simulink model "Problem8"  (R2020b)
settings: Solver=VariableStepAuto  StartTime=0.0  StopTime=inf  RelTol=1e-3
settings Model: Creator=Dell  LastModifiedBy=Dell

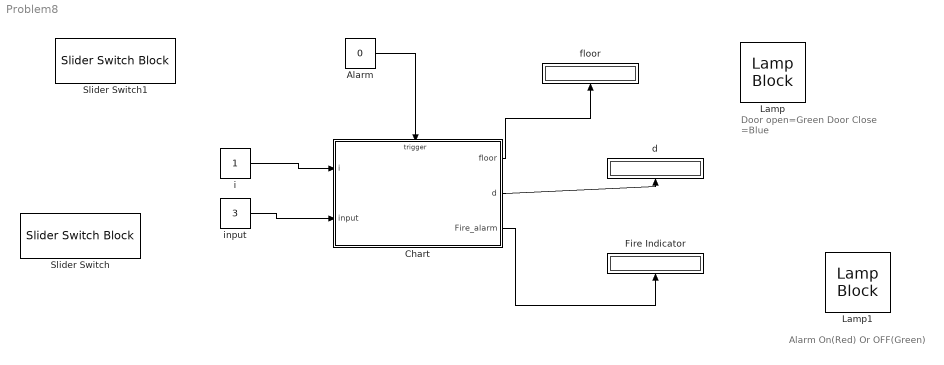
== system Problem8 ==
  note: Alarm On(Red) Or OFF(Green)
  note: Door open=Green
      | Door Close =Blue
  Alarm : Constant  Value=0
  Chart : Stateflow chart  TreatAsAtomicUnit=on
  Fire Indicator : Display
  Lamp : LampBlock
  Lamp1 : LampBlock
  Slider Switch : SliderSwitchBlock
      settings: Values={{'Off', 'On'}, [0 1]}
  Slider Switch1 : SliderSwitchBlock
      settings: Values={{'Off', 'On'}, [0 1]}
  d : Display
  floor : Display
  i : Constant
  input : Constant  Value=3
  wires:
  Chart/1(floor) -> floor/1
  input/1 -> Chart/2(input)
  i/1 -> Chart/1(i)
  Chart/2(d) -> d/1
  Alarm/1 -> Chart/Trigger
  Chart/3(Fire_alarm) -> Fire Indicator/1

== stateflow chart Problem8/Chart ==
  settings: executeAtInitialization=1
  state Close
    d=1;
    state f2
      floor=2;
    state f3
      floor=3;
    state f4
      floor=4;
    state G
      floor=0;
    state f1
      floor=1;
    (default) -> G
    f2 -> f3 : [ input==3|| input==4]
    f3 -> f4 : [input==4]
    f1 -> f2 : [input==2 || input==3|| input==4]
    G -> f1 : [input==1 || input==2 || input==3|| input==4]
  state open
    d=0;
  (default) -> Close
  open -> Close : [i==1]
  Close -> open [order 1] : [i==0]
  (junction 152) -> open [order 2]
  Close -> (junction 152) [order 2]
  (junction 152) -> (junction 159) [order 1] : Alarm{Fire_alarm=1}
  data: i input; input input; floor output; d output; Fire_alarm output
  events: Alarm input RISING_EDGE_EVENT
